simulink model "omega_input"  (Simulink 10.1)
settings: Solver=VariableStepAuto  StartTime=0.0  StopTime=2.0  RelTol=1e-3
undefined symbols (not defined in the file): inner_h, omega_max_lim, omega_min_lim, sample_time
libraries: simulink x3
settings Model: Creator=martinhe  LastModifiedBy=martinhe
settings DataIOCC: SaveFormat=Dataset  ReturnWorkspaceOutputs=on
settings OptimizationCC: LifeSpan=auto
settings DebuggingCC: UnderspecifiedInitializationDetection=Simplified  MergeDetectMultiDrivingBlocksExec=error  SFUnexpectedBacktrackingDiag=error  SFNoUnconditionalDefaultTransitionDiag=error  SFExecutionAtInitializationDiag=warning  ArithmeticOperatorsInVariantConditions=error
settings HardwareCC: ProdBitPerPointer=64  ProdBitPerSizeT=64  ProdBitPerPtrDiffT=64  ProdLargestAtomicFloat=Float  ProdIntDivRoundTo=Zero  ProdEndianess=LittleEndian  ProdWordSize=64  ProdHWDeviceType=Intel->x86-64 (Windows64)
settings ModelReferenceCC: PropagateSignalLabelsOutOfModel=on
settings SFSimCC: SimUseLocalCustomCode=on  CustomCodeUndefinedFunction=FilterOut
settings RTWCC: RTWUseLocalCustomCode=on
settings CodeAppCC: StateflowObjectComments=off
settings GRTTargetCC: TargetLangStandard=C99 (ISO)  CombineOutputUpdateFcns=on  GRTInterface=off
settings ConfigComp: CovMetricSettings=dwe  CovHtmlReporting=off  CovSaveCumulativeToWorkspaceVar=off  CovSaveSingleToWorkspaceVar=off  CovExternalEMLEnable=on

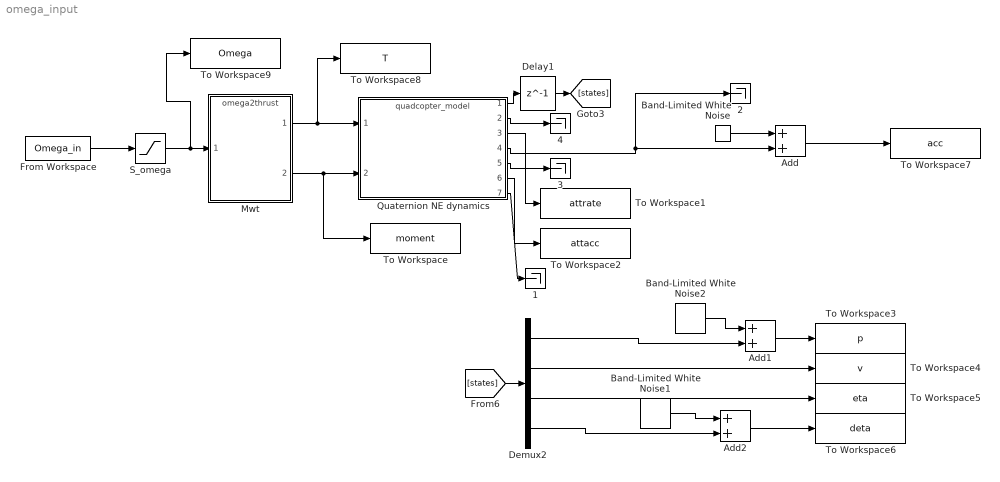
== system omega_input ==
     {1..4} (4 alike) : Terminator
  Add : Sum
  Add1 : Sum
  Add2 : Sum
  Band-Limited White Noise : simulink/Sources/Band-Limited White Noise  Cov=acc_noise_power  Ts=inner_h  seed=[23341]
  Band-Limited White Noise1 : simulink/Sources/Band-Limited White Noise  Cov=deta_noise_power  Ts=inner_h  seed=[23341]
  Band-Limited White Noise2 : simulink/Sources/Band-Limited White Noise  Cov=p_noise_power  Ts=inner_h  seed=[23341]
  Delay1 : Delay  DelayLength=1  SampleTime=inner_h
  Demux2 : Demux  Outputs=[3,3,3,3]
  From Workspace : FromWorkspace  VariableName=Omega_in
  Mwt : ModelReference  ModelNameDialog=omega2thrust.mdl  SimulationMode=Normal  ModelReferenceVersion=1.5
  Quaternion NE dynamics : ModelReference  ModelNameDialog=quadcopter_model.mdl  SimulationMode=Normal  ModelReferenceVersion=1.341
  S_omega : Saturate  UpperLimit=omega_max_lim  LowerLimit=omega_min_lim
  To Workspace : ToWorkspace  VariableName=moment  SaveFormat=Timeseries  SampleTime=sample_time
  To Workspace1 : ToWorkspace  VariableName=attrate  SaveFormat=Timeseries  SampleTime=sample_time
  To Workspace2 : ToWorkspace  VariableName=attacc  SaveFormat=Timeseries  SampleTime=sample_time
  To Workspace3 : ToWorkspace  VariableName=p  SaveFormat=Timeseries  SampleTime=sample_time
  To Workspace4 : ToWorkspace  VariableName=v  SaveFormat=Timeseries  SampleTime=sample_time
  To Workspace5 : ToWorkspace  VariableName=eta  SaveFormat=Timeseries  SampleTime=sample_time
  To Workspace6 : ToWorkspace  VariableName=deta  SaveFormat=Timeseries  SampleTime=sample_time
  To Workspace7 : ToWorkspace  VariableName=acc  SaveFormat=Timeseries  SampleTime=sample_time
  To Workspace8 : ToWorkspace  VariableName=T  SaveFormat=Timeseries  SampleTime=sample_time
  To Workspace9 : ToWorkspace  VariableName=Omega  SaveFormat=Timeseries  SampleTime=sample_time
  wires:
  Quaternion NE dynamics/6 -> To Workspace2/1
  Quaternion NE dynamics/1 -> Delay1/1
  Quaternion NE dynamics/5 -> "   3"/1
  Quaternion NE dynamics/2 -> "   4"/1
  Delay1/1 -> [states]
  S_omega/1 -> To Workspace9/1, Mwt/1
  Quaternion NE dynamics/3 -> To Workspace1/1
  Quaternion NE dynamics/4 -> Add/2, "   2"/1
  Mwt/1 -> To Workspace8/1, Quaternion NE dynamics/1
  Mwt/2 -> To Workspace/1, Quaternion NE dynamics/2
  From Workspace/1 -> S_omega/1
  Demux2/2 -> To Workspace4/1
  Demux2/3 -> To Workspace5/1
  [states] -> Demux2/1
  Add/1 -> To Workspace7/1
  Band-Limited White Noise/1 -> Add/1
  Add1/1 -> To Workspace3/1
  Demux2/1 -> Add1/2
  Band-Limited White Noise2/1 -> Add1/1
  Add2/1 -> To Workspace6/1
  Demux2/4 -> Add2/2
  Band-Limited White Noise1/1 -> Add2/1
  Quaternion NE dynamics/7 -> "   1"/1
